simulink model "quadcopter_rotation_subsystem"  (R2023b)
settings: Solver=ode3  StartTime=0  StopTime=inf  FixedStep=0.005  RelTol=1e-3  EnableMultiTasking=on
values from neighbouring files (symbols this model uses):
  alpha_vect = A\B    [poly3traj.m]
  g = 9.81    [MRB.m]
  Ic = [Ixx,0,0;0,Iyy,0;0,0,Izz]    [MRB.m]
  m = 4    [MRB.m]
  Mrb = [m*eye(3),zeros(3);zeros(3),Ic]    [MRB.m]
libraries: aerolibutil x11, simulink_extras x10, slpidlib x6, sharedtransform x3, sharedutil x2, vrlib x2
(part 2 of 2)

== system quadcopter_rotation_subsystem/Formatting/Euler to VR/Quaternion Normalization2 ==
  e0 : Inport
  1/2 : Gain  Gain=1/2  SaturateOnIntegerOverflow=on  OutDataTypeStr=Inherit: Same as input  ParamDataTypeStr=Inherit: Same as input
  Demux : Demux  Outputs=[1 3]
      settings: DisplayOption=none
  Mux : Mux  Inputs=2
  Product : Product  InputSameDT=on  SaturateOnIntegerOverflow=on  OutDataTypeStr=Inherit: Same as first input
  Trigonometric Function : Trigonometry
  Trigonometric Function1 : Trigonometry  Operator=cos
  e0_norm : Outport  VectorParamsAs1DForOutWhenUnconnected=off
  wires:
  Trigonometric Function1/1 -> Mux/1
  Demux/2 -> Product/2
  Demux/1 -> 1/2/1
  Mux/1 -> e0_norm/1
  Product/1 -> Mux/2
  Trigonometric Function/1 -> Product/1
  1/2/1 -> Trigonometric Function1/1, Trigonometric Function/1
  e0/1 -> Demux/1

== system quadcopter_rotation_subsystem/Mathematical model/Enabled Subsystem/Subsystem ==
  vector : Inport
  vector1 : Inport  Port=2
  " generateQ" : MATLAB Function  TreatAsAtomicUnit=on
  RotateMatrix : MATLAB Function  TreatAsAtomicUnit=on
  Switch : Switch  Criteria=u2 > Threshold  Threshold=7  SaturateOnIntegerOverflow=off  InputSameDT=off
  generate value : MATLAB Function  Commented=on  TreatAsAtomicUnit=on
  reverseQ : MATLAB Function  TreatAsAtomicUnit=on
  original_vector : Outport
  wires:
  vector/1 -> RotateMatrix/2(vector)
  " generateQ"/1(q) -> reverseQ/1(q), RotateMatrix/1(q)
  RotateMatrix/1(rotated_vector) -> reverseQ/2(vector), Switch/3
  Switch/1 -> original_vector/1
  vector1/1 -> Switch/2
  reverseQ/1(original_vector) -> Switch/1

== system quadcopter_rotation_subsystem/Mathematical model/Enabled Subsystem1/rotation system ==
  time_step : Inport
  Product1 : Product
  Quaternion Inverse : aerolibutil/Quaternion Inverse
  "Quaternion rotation " : Subsystem
  RotateMatrix : MATLAB Function  Commented=on  TreatAsAtomicUnit=on
  Switch : Switch  Criteria=u2 > Threshold  Threshold=7  SaturateOnIntegerOverflow=off  InputSameDT=off
  generate value : MATLAB Function  Commented=on  TreatAsAtomicUnit=on
  k : Constant  Value=[1;0;0]  VectorParams1D=off
  reverseQ : MATLAB Function  Commented=on  TreatAsAtomicUnit=on
  q : Outport
  wires:
  "Quaternion rotation "/1(q rotation) -> Product1/1, Quaternion Inverse/1, Switch/3
  Switch/1 -> q/1
  Product1/1 -> Switch/1
  k/1 -> "Quaternion rotation "/1(axis vector rotation)
  time_step/1 -> Switch/2, "Quaternion rotation "/2(t)
  Quaternion Inverse/1 -> Product1/2

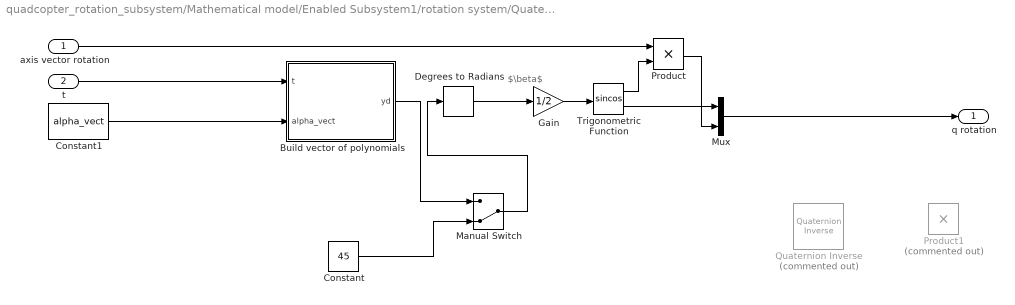
== system quadcopter_rotation_subsystem/Mathematical model/Enabled Subsystem1/rotation system/Quaternion rotation  ==
  note: $\beta$
  axis vector rotation : Inport
  t : Inport  Port=2
  Build vector of polynomials : MATLAB Function  TreatAsAtomicUnit=on
  Constant : Constant  Value=45
  Constant1 : Constant  Value=alpha_vect  VectorParams1D=off
  Degrees to Radians : simulink_extras/Transformations/Degrees to Radians
  Gain : Gain  Gain=1/2
  Manual Switch : ManualSwitch  CurrentSetting=0
  Mux : Mux  Inputs=2
  Product : Product
  Product1 : Product  Commented=on
  Quaternion Inverse : aerolibutil/Quaternion Inverse  Commented=on
  Trigonometric Function : Trigonometry  Operator=sincos
  q rotation : Outport
  wires:
  Gain/1 -> Trigonometric Function/1
  Trigonometric Function/2 -> Mux/1
  axis vector rotation/1 -> Product/1
  Degrees to Radians/1 -> Gain/1
  Trigonometric Function/1 -> Product/2
  Constant1/1 -> Build vector of polynomials/2(alpha_vect)
  Product/1 -> Mux/2
  Mux/1 -> q rotation/1
  t/1 -> Build vector of polynomials/1(t)
  Constant/1 -> Manual Switch/2
  Build vector of polynomials/1(yd) -> Manual Switch/1
  Manual Switch/1 -> Degrees to Radians/1

== matlab function quadcopter_rotation_subsystem/Mathematical model/Enabled Subsystem1/rotation system/reverseQ ==
  data: q input; original_vector output; vector input
function original_vector = revertQuaternionRotation(q, vector)
    % Extract quaternion components
    w = q(1);
    x = -q(2);
    y = -q(3);
    z = -q(4);
    % Inverse quaternion (conjugate for unit quaternion)
    % Apply inverse rotation
     % Quaternion rotation matrix again but with the inverse quartonion
     % this time
    R = [1 - 2*y^2 - 2*z^2, 2*x*y - 2*z*w, 2*x*z + 2*y*w;
         2*x*y + 2*z*w, 1 - 2*x^2 - 2*z^2, 2*y*z - 2*x*w;
         2*x*z - 2*y*w, 2*y*z + 2*x*w, 1 - 2*x^2 - 2*y^2];
    % Apply rotation on the inverse
    original_vector = R * vector;
end

== matlab function quadcopter_rotation_subsystem/Flight Control System/Outer loop position control/MATLAB Function ==
  data: Deltap_e input; Deltap_b output; psi input
function Deltap_b = fcn(Deltap_e,psi)

R = [ cos(psi) , -sin(psi) ;
      sin(psi) ,  cos(psi) ];

Deltap_b = R'*Deltap_e;

== matlab function quadcopter_rotation_subsystem/Mathematical model/scaled time 1 ==
  data: t1 input; counter_timer input; t2 output; counter_timer output
function [t2,counter_timer] = fcn(t1,counter_timer)
 
if t1 == counter_timer(2)
   counter_timer(1) = counter_timer(1) +1; 
   counter_timer(2) = counter_timer(2) + 2.5;
      
end
if counter_timer(1) == 11
  counter_timer(1) = 0;
end

t2 = counter_timer(1);

== matlab function quadcopter_rotation_subsystem/Mathematical model/ memory block ==
  data: q input; q2 output; counter input; counter output
function [q2,counter] = fcn(q,counter)
t = floor(q(1)*10000);
tc = floor(counter*10000);

if q ==  [0; 0; 0; 0] 
    q = [1 ;0; 0; 0];
end
disp(q);

if t == 8535 
 q = [1 ;0; 0; 0];
 counter = q(1);
end

if t == 9240 && tc == 8535

  q = [1 ;0; 0; 0];
  counter = q(1);

end
q2 = q;

== matlab function quadcopter_rotation_subsystem/Mathematical model/Rigid-body dynamics/MATLAB Function ==
  data: nu input; Cnunu output; m input; Ic input
function Cnunu = fcn(nu,m,Ic)

v = nu(1:3);  % linear velocities (expressed in the body frame)
omega = nu(4:6); % angular velocities (expressed in the body frame)

% Coriolis term
Cnunu = [ cross(omega,m*v) ; -cross(Ic*omega,omega) ];

== matlab function quadcopter_rotation_subsystem/Mathematical model/Quaternion rotation /Build vector of polynomials ==
  data: t input; yd output; alpha_vect input
function yd = fcn(t,alpha_vect)


    t_vect0 = [ 1 ; t ; t^2 ; t^3 ; t^4 ; t^5 ]; % vector of t values
    %t_vect0 = [ 1 ; t ; t^2 ; t^3 ]; % vector of t values


yd = t_vect0'*alpha_vect;

== matlab function quadcopter_rotation_subsystem/Build vector of polynomials ==
  data: t input; yd output; alpha_vect input
function yd = fcn(t,alpha_vect)

    %t_vect0 = [ 1 ; t ; t^2 ; t^3 ; t^4 ; t^5 ]; % vector of t values
    t_vect0 = [1; t; t^2; t^3];  % vector of t values for cubic polynomial
 
yd = t_vect0'*alpha_vect;

== matlab function quadcopter_rotation_subsystem/Mathematical model/Enabled Subsystem1/rotation system/Quaternion rotation /Build vector of polynomials ==
  data: t input; yd output; alpha_vect input
function yd = fcn(t,alpha_vect)


    t_vect0 = [ 1 ; t ; t^2 ; t^3 ; t^4 ; t^5 ]; % vector of t values
    %t_vect0 = [ 1 ; t ; t^2 ; t^3 ]; % vector of t values


yd = t_vect0'*alpha_vect;

== matlab function quadcopter_rotation_subsystem/Mathematical model/Enabled Subsystem/Subsystem/ generateQ ==
  data: q output
function q = generateQuaternion()
    %angle in radians (45 degrees) or beta
    angle_radians = deg2rad(45);
    % Fixed axis 
    axis = [1; 0; 0];
    % Calculate the quaternion
    q = [cos(angle_radians / 2); sin(angle_radians / 2) * axis];
end

== matlab function quadcopter_rotation_subsystem/Mathematical model/Enabled Subsystem/Subsystem/RotateMatrix ==
  data: q input; rotated_vector output; vector input
function rotated_vector = applyQuaternionRotation(q, vector)
    % quaternion components
    w = q(1);
    x = q(2);
    y = q(3);
    z = q(4);
    % Quaternion rotation matrix
    R = [1 - 2*y^2 - 2*z^2, 2*x*y - 2*z*w, 2*x*z + 2*y*w;
         2*x*y + 2*z*w, 1 - 2*x^2 - 2*z^2, 2*y*z - 2*x*w;
         2*x*z - 2*y*w, 2*y*z + 2*x*w, 1 - 2*x^2 - 2*y^2];
    % rotate
    rotated_vector = R * vector;
end

== matlab function quadcopter_rotation_subsystem/Mathematical model/Enabled Subsystem/Subsystem/generate value ==
  data: y output
function y = random_counter()
    persistent counter;
    
    % Initialize counter if not already initialized
    if isempty(counter)
        counter = 0;
    end
    
    % Increment counter
    counter = counter + 1;
    display(counter)
    % Check if counter has reached a random interval between 0 and 20
    if counter >= 2
        
        % Reset counter to 0
        counter = 0;
    end
    
    y = counter;
end

== matlab function quadcopter_rotation_subsystem/Mathematical model/Enabled Subsystem/Subsystem/reverseQ ==
  data: q input; original_vector output; vector input
function original_vector = revertQuaternionRotation(q, vector)
    % Extract quaternion components
    w = q(1);
    x = -q(2);
    y = -q(3);
    z = -q(4);
    % Inverse quaternion (conjugate for unit quaternion)
    % Apply inverse rotation
     % Quaternion rotation matrix again but with the inverse quartonion
     % this time
    R = [1 - 2*y^2 - 2*z^2, 2*x*y - 2*z*w, 2*x*z + 2*y*w;
         2*x*y + 2*z*w, 1 - 2*x^2 - 2*z^2, 2*y*z - 2*x*w;
         2*x*z - 2*y*w, 2*y*z + 2*x*w, 1 - 2*x^2 - 2*y^2];
    % Apply rotation on the inverse
    original_vector = R * vector;
end

== matlab function quadcopter_rotation_subsystem/Mathematical model/scaled time  ==
  data: u input; counter_timer input; y output; counter_timer output
function [y,counter_timer] = fcn(u,counter_timer)
 
if u == counter_timer(2)
   counter_timer(1) = counter_timer(1) +1; 
   counter_timer(2) = counter_timer(2) + 25;
      
end
if counter_timer(1) == 11
  counter_timer(1) = 0;
end

y = counter_timer(1);

== matlab function quadcopter_rotation_subsystem/Mathematical model/Enabled Subsystem1/rotation system/RotateMatrix ==
  data: q input; rotated_vector output; vector input
function rotated_vector = applyQuaternionRotation(q, vector)
    % quaternion components
    w = q(1);
    x = q(2);
    y = q(3);
    z = q(4);
    % Quaternion rotation matrix
    R = [1 - 2*y^2 - 2*z^2, 2*x*y - 2*z*w, 2*x*z + 2*y*w;
         2*x*y + 2*z*w, 1 - 2*x^2 - 2*z^2, 2*y*z - 2*x*w;
         2*x*z - 2*y*w, 2*y*z + 2*x*w, 1 - 2*x^2 - 2*y^2];
    % rotate
    rotated_vector = R * vector;
end

== matlab function quadcopter_rotation_subsystem/Mathematical model/Enabled Subsystem1/rotation system/generate value ==
  data: y output
function y = random_counter()
    persistent counter;
    
    % Initialize counter if not already initialized
    if isempty(counter)
        counter = 0;
    end
    
    % Increment counter
    counter = counter + 1;
    display(counter)
    % Check if counter has reached a random interval between 0 and 20
    if counter >= 2
        
        % Reset counter to 0
        counter = 0;
    end
    
    y = counter;
end
